simulink subsystem "Trajectory"  (R2021a)
settings: Solver=VariableStepAuto  StartTime=0.0  StopTime=10.0  RelTol=1e-3
undefined symbols (not defined in the file): DiscIntNeverNeededParam, MPC, mpc
libraries: robotlib x5, sharedtransform x2, robotcorelib x2, eeGeneralControl x1
settings Model: Creator=Lamarre  LastModifiedBy=lamarre
settings SolverCC: AlgebraicLoopSolver=TrustRegion
settings DebuggingCC: SFMachineParentedDataDiag=warning

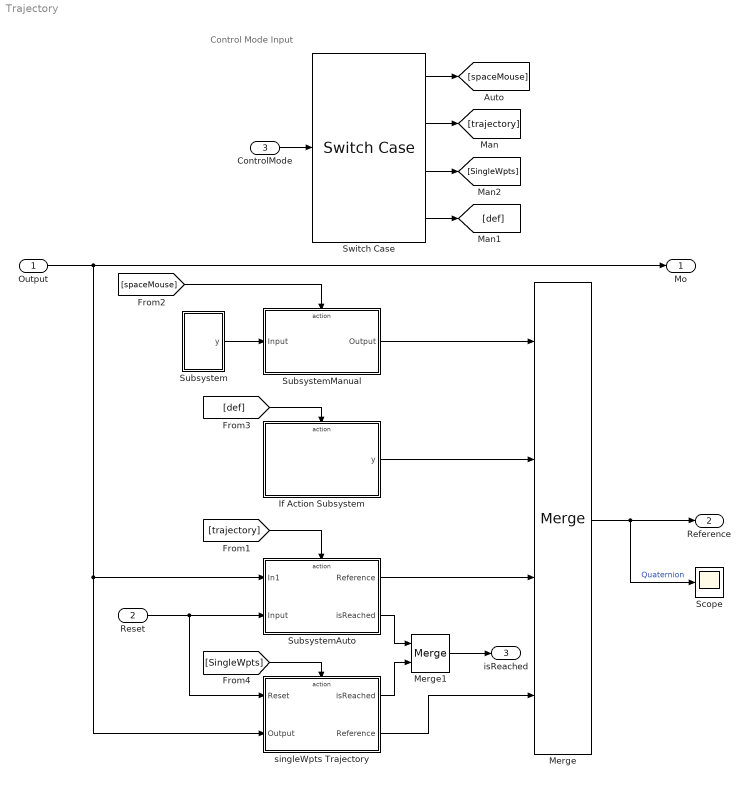
== system Trajectory ==
  note: Control Mode Input
  Output : Inport
  Reset : Inport  Port=2
  ControlMode : Inport  Port=3
  If Action Subsystem : Subsystem  TreatAsAtomicUnit=on
  Merge : Merge  Inputs=4
  Merge1 : Merge
  Scope : Scope
  Subsystem : Subsystem
  SubsystemAuto : Subsystem
  SubsystemManual : Subsystem
  Switch Case : SwitchCase  CaseConditions={mode.traj.SpaceMouseMode,mode.traj.trajMode, mode.traj.singleWpts,}
  singleWpts Trajectory : Subsystem
  Mo : Outport
  Reference : Outport  Port=2
  isReached : Outport  Port=3
  wires:
  Output/1 -> SubsystemAuto/1(In1), singleWpts Trajectory/2(Output), Mo/1
  Reset/1 -> SubsystemAuto/2(Input), singleWpts Trajectory/1(Reset)
  ControlMode/1 -> Switch Case/1
  [trajectory] -> SubsystemAuto/Action
  SubsystemManual/1(Output) -> Merge/1
  Subsystem/1(y) -> SubsystemManual/1(Input)
  [spaceMouse] -> SubsystemManual/Action
  Merge/1 -> Reference/1, Scope/1  "Quaternion"
  Switch Case/1 -> [spaceMouse]
  Switch Case/2 -> [trajectory]
  [def] -> If Action Subsystem/Action
  If Action Subsystem/1(y) -> Merge/2
  Switch Case/4 -> [def]
  Switch Case/3 -> [SingleWpts]
  [SingleWpts] -> singleWpts Trajectory/Action
  SubsystemAuto/2(isReached) -> Merge1/1
  Merge1/1 -> isReached/1
  singleWpts Trajectory/1("isReached ") -> Merge1/2
  singleWpts Trajectory/2("Reference ") -> Merge/4
  SubsystemAuto/1(Reference) -> Merge/3

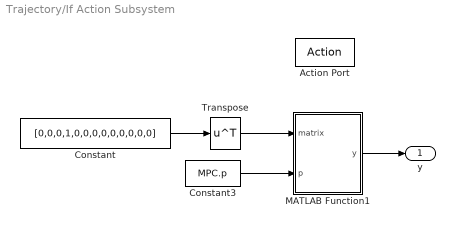
== system Trajectory/If Action Subsystem ==
  Action Port : ActionPort
  Constant : Constant  Value=[0,0,0,1,0,0,0,0,0,0,0,0,0]
  Constant3 : Constant  Value=MPC.p
  MATLAB Function1 : MATLAB Function  TreatAsAtomicUnit=on
  Transpose : Math  Operator=transpose  OutputSignalType=real  SaturateOnIntegerOverflow=on
  y : Outport
  wires:
  Constant/1 -> Transpose/1
  MATLAB Function1/1(y) -> y/1
  Constant3/1 -> MATLAB Function1/2(p)
  Transpose/1 -> MATLAB Function1/1(matrix)

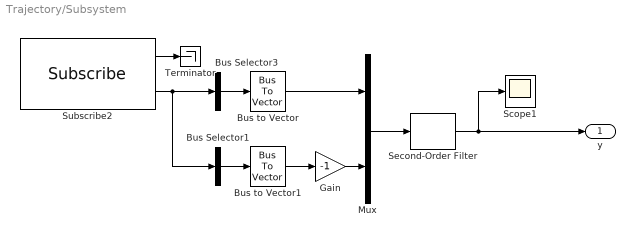
== system Trajectory/Subsystem ==
  Bus Selector1 : BusSelector  OutputSignals=Angular.X,Angular.Y,Angular.Z  OutputAsBus=on
  Bus Selector3 : BusSelector  OutputSignals=Linear.X,Linear.Y,Linear.Z  OutputAsBus=on
  Bus to Vector : BusToVector
  Bus to Vector1 : BusToVector
  Gain : Gain  Gain=-1
  Mux : Mux  Inputs=2
  Scope1 : Scope
  Second-Order Filter : eeGeneralControl/Second-Order Filter  FilterType=Low-pass  fn=wn_l  Zeta=zeta_l  Ts=1/25  A0=0  Ph0=0  f0=0  b0=0
      settings: SourceProductBaseCode=PS
  Subscribe2 : robotlib/Subscribe  topicSource=Specify your own  topic=/spacenav/twist  messageType=geometry_msgs/Twist  SampleTime=1/25  legacyBusStruct=off  messageQueueLength=2
  Terminator : Terminator
  y : Outport
  wires:
  Mux/1 -> Second-Order Filter/1
  Bus to Vector/1 -> Mux/1
  Gain/1 -> Mux/2
  Bus to Vector1/1 -> Gain/1
  Bus Selector1/1 -> Bus to Vector1/1
  Bus Selector3/1 -> Bus to Vector/1
  Subscribe2/1 -> Terminator/1
  Subscribe2/2 -> Bus Selector3/1, Bus Selector1/1
  Second-Order Filter/1 -> Scope1/1, y/1

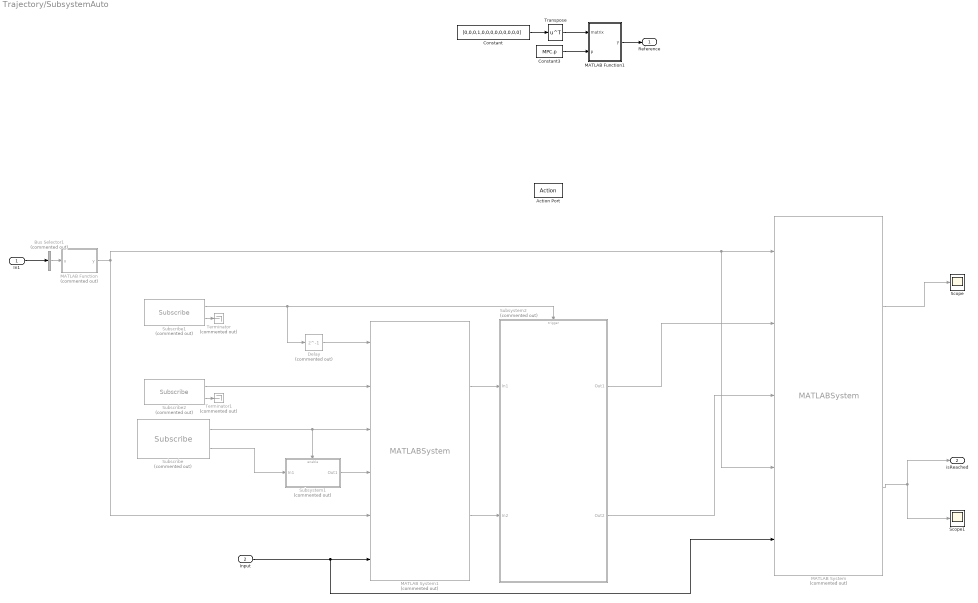
== system Trajectory/SubsystemAuto ==
  In1 : Inport
  Input : Inport  Port=2
  Action Port : ActionPort
  Bus Selector1 : BusSelector  Commented=on  OutputSignals=World Position,qS2W  OutputAsBus=on
  Constant : Constant  Value=[0,0,0,1,0,0,0,0,0,0,0,0,0]
  Constant3 : Constant  Value=MPC.p
  Delay : Delay  Commented=on  DelayLength=1
  MATLAB Function : MATLAB Function  Commented=on  TreatAsAtomicUnit=on
  MATLAB Function1 : MATLAB Function  TreatAsAtomicUnit=on
  MATLAB System : MATLABSystem  Commented=on  System=TrajectoryManager  SampleTime=mpc.Ts  OffsetTime=0  prediction=mpc.p  bufferSize=6001  linearConvergence=.2  quaternionConvergence=.1  TargetThreshold=3  SimulateUsing=Code generation
      mask Type: TrajectoryManager
      mask Display:
      | disp('TrajectoryManager');
      | port_label('input',1,'mesuredPose');
      | port_label('input',2,'poses');
      | port_label('input',3,'isNew');
      | port_label('input',4,'x0');
      | port_label('input',5,'reset');
      | port_label('output',1,'currentPose');
      | port_label('output',2,'isReached');
  MATLAB System1 : MATLABSystem  Commented=on  System=AddPose  buffSize=20  elementSize=8  SimulateUsing=Interpreted execution
      mask Type: AddPose
      mask Display:
      | disp('AddPose');
      | port_label('input',1,'compute');
      | port_label('input',2,'clearBuffer');
      | port_label('input',3,'isNew');
      | port_label('input',4,'waypoint');
      | port_label('input',5,'initCond');
      | port_label('input',6,'reset');
      | port_label('output',1,'waypoints');
      | port_label('output',2,'count');
  Scope : Scope
  Scope1 : Scope
  Subscribe : robotlib/Subscribe  Commented=on  topicSource=Specify your own  topic=proc_control/add_pose  messageType=sonia_common/AddPose  SampleTime=-1  legacyBusStruct=off  messageQueueLength=1
      link override SourceBlock: ROSTopic=/my_topic  ROSMessageType=geometry_msgs/Point  SLBusName=SL_Bus_Test_Traj_geometry_msgs_Point  ModelName=Test_Traj  BlockId=Sub_Test_Traj_124
  Subscribe1 : robotlib/Subscribe  Commented=on  topicSource=Specify your own  topic=/proc_control/compute_trajectory  messageType=std_msgs/Bool  SampleTime=-1  legacyBusStruct=off  messageQueueLength=1
  Subscribe2 : robotlib/Subscribe  Commented=on  topicSource=Specify your own  topic=/proc_control/clear_waypoints  messageType=std_msgs/Bool  SampleTime=-1  legacyBusStruct=off  messageQueueLength=1
  Subsystem1 : Subsystem  Commented=on
  Subsystem2 : Subsystem  Commented=on
  Terminator : Terminator  Commented=on
  Terminator1 : Terminator  Commented=on
  Transpose : Math  Operator=transpose  OutputSignalType=real  SaturateOnIntegerOverflow=on
  Reference : Outport
  isReached : Outport  Port=2
  wires:
  Constant/1 -> Transpose/1
  Constant3/1 -> MATLAB Function1/2(p)
  Transpose/1 -> MATLAB Function1/1(matrix)
  MATLAB Function1/1(y) -> Reference/1
  Subscribe2/2 -> Terminator1/1
  Subscribe1/2 -> Terminator/1
  Input/1 -> MATLAB System1/6, MATLAB System/5
  Subscribe2/1 -> MATLAB System1/2
  MATLAB Function/1(y) -> MATLAB System1/5, MATLAB System/1, MATLAB System/4
  Subscribe/1 -> MATLAB System1/3, Subsystem1/Enable
  MATLAB System/1 -> Scope/1
  Subsystem2/1(Out1) -> MATLAB System/2
  Subsystem2/2(Out2) -> MATLAB System/3
  Subscribe/2 -> Subsystem1/1(In1)
  Subsystem1/1(Out1) -> MATLAB System1/4
  In1/1 -> Bus Selector1/1
  MATLAB System/2 -> Scope1/1, isReached/1
  MATLAB System1/2 -> Subsystem2/2(In2)
  Subscribe1/1 -> Delay/1, Subsystem2/Trigger
  Bus Selector1/1 -> MATLAB Function/1(u)
  MATLAB System1/1 -> Subsystem2/1(In1)
  Delay/1 -> MATLAB System1/1

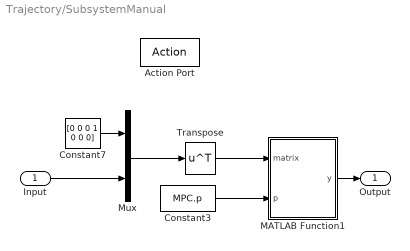
== system Trajectory/SubsystemManual ==
  Input : Inport
  Action Port : ActionPort
  Constant3 : Constant  Value=MPC.p
  Constant7 : Constant  Value=[0 0 0 1 0 0 0]
  MATLAB Function1 : MATLAB Function  TreatAsAtomicUnit=on
  Mux : Mux  Inputs=2
  Transpose : Math  Operator=transpose  OutputSignalType=real  SaturateOnIntegerOverflow=on
  Output : Outport
  wires:
  MATLAB Function1/1(y) -> Output/1
  Mux/1 -> Transpose/1
  Constant3/1 -> MATLAB Function1/2(p)
  Transpose/1 -> MATLAB Function1/1(matrix)
  Input/1 -> Mux/2
  Constant7/1 -> Mux/1

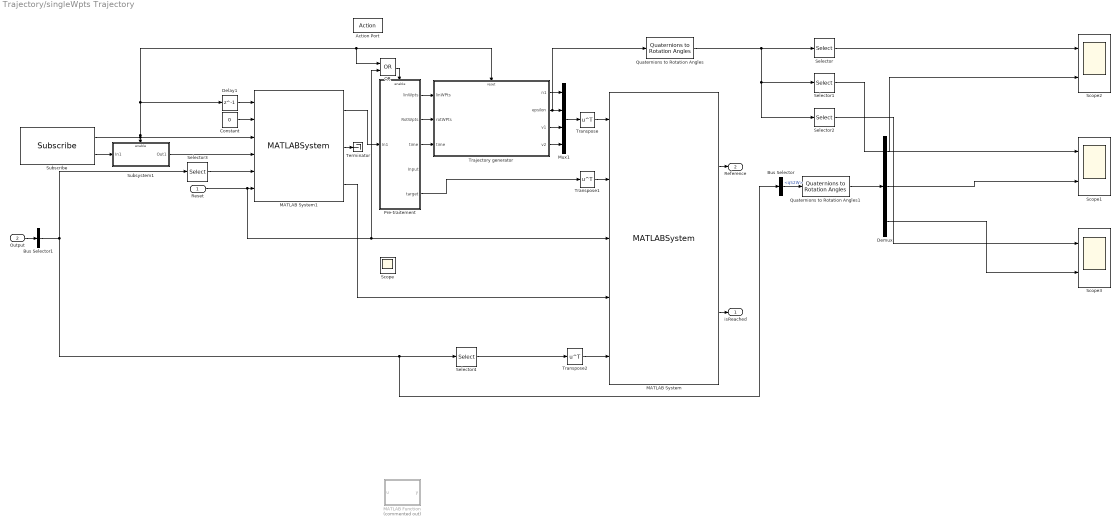
== system Trajectory/singleWpts Trajectory ==
  Reset : Inport
  Output : Inport  Port=2
  Action Port : ActionPort  InitializeStates=reset
  Bus Selector : BusSelector  OutputSignals=qS2W
  Bus Selector1 : BusSelector  OutputSignals=World Position,qS2W,Body Velocity,Angular Rate  OutputAsBus=on
  Constant : Constant  Value=0
  Delay1 : Delay  DelayLength=1
  Demux : Demux  Outputs=3
  MATLAB Function : MATLAB Function  Commented=on  TreatAsAtomicUnit=on
  MATLAB System : MATLABSystem  System=TrajectoryManager  SampleTime=MPC.Ts  OffsetTime=0  prediction=MPC.p  bufferSize=6001  linearConvergence=.25  quaternionConvergence=.22  TargetThreshold=2  SimulateUsing=Code generation
      mask Type: TrajectoryManager
      mask Display:
      | disp('TrajectoryManager');
      | port_label('input',1,'poses');
      | port_label('input',2,'target');
      | port_label('input',3,'reset');
      | port_label('input',4,'x0');
      | port_label('input',5,'mesuredPose');
      | port_label('output',1,'currentPose');
      | port_label('output',2,'isReached');
  MATLAB System1 : MATLABSystem  System=AddPose  buffSize=2  elementSize=9  SimulateUsing=Code generation
      mask Type: AddPose
      mask Display:
      | disp('AddPose');
      | port_label('input',1,'compute');
      | port_label('input',2,'clearBuffer');
      | port_label('input',3,'isNew');
      | port_label('input',4,'waypoint');
      | port_label('input',5,'xk');
      | port_label('input',6,'reset');
      | port_label('output',1,'waypoints');
      | port_label('output',2,'count');
      | port_label('output',3,'initCond');
  Mux1 : Mux
  OR : Logic  Operator=OR  AllPortsSameDT=off  OutDataTypeStr=boolean
  Pre-traitement : Subsystem
  Quaternions to Rotation Angles : sharedtransform/Quaternions to Rotation Angles  rotationOrder=ZYX  aMode=aMode
      settings: SourceProductBaseCode=AE,PW,DR,MT,UV,VE
  Quaternions to Rotation Angles1 : sharedtransform/Quaternions to Rotation Angles  rotationOrder=ZYX  aMode=aMode
      settings: SourceProductBaseCode=AE,PW,DR,MT,UV,VE
  Scope : Scope
  Scope1 : Scope  NumInputPorts=2
  Scope2 : Scope  NumInputPorts=2
  Scope3 : Scope  NumInputPorts=2
  Selector : Selector  InputPortWidth=3  IndexOptions=Index vector (dialog)  Indices=[1]  OutputSizes=1
  Selector1 : Selector  InputPortWidth=3  IndexOptions=Index vector (dialog)  Indices=[2]  OutputSizes=1
  Selector2 : Selector  InputPortWidth=3  IndexOptions=Index vector (dialog)  Indices=[3]  OutputSizes=1
  Selector3 : Selector  InputPortWidth=13  IndexOptions=Index vector (dialog)  Indices=[1:7]  OutputSizes=1
  Selector4 : Selector  InputPortWidth=13  IndexOptions=Index vector (dialog)  Indices=[1:13]  OutputSizes=1
  Subscribe : robotlib/Subscribe  topicSource=Specify your own  topic=proc_control/add_pose  messageType=sonia_common/AddPose  SampleTime=-1  legacyBusStruct=off  messageQueueLength=1
      link override SourceBlock: ROSTopic=/my_topic  ROSMessageType=geometry_msgs/Point  SLBusName=SL_Bus_Test_Traj_geometry_msgs_Point  ModelName=Test_Traj  BlockId=Sub_Test_Traj_124
  Subsystem1 : Subsystem
  Terminator : Terminator
  Trajectory generator : Subsystem
  Transpose : Math  Operator=transpose  SaturateOnIntegerOverflow=on
  Transpose1 : Math  Operator=transpose  SaturateOnIntegerOverflow=on
  Transpose2 : Math  Operator=transpose  SaturateOnIntegerOverflow=on
  "isReached " : Outport
  "Reference " : Outport  Port=2
  wires:
  Bus Selector/1 -> Quaternions to Rotation Angles1/1  "<qS2W>"
  Quaternions to Rotation Angles1/1 -> Demux/1
  Quaternions to Rotation Angles/1 -> Selector/1, Selector1/1, Selector2/1
  Trajectory generator/2(epsilon) -> Mux1/2, Quaternions to Rotation Angles/1
  Transpose2/1 -> MATLAB System/5
  MATLAB System1/3 -> MATLAB System/4
  Transpose1/1 -> MATLAB System/2
  Pre-traitement/5(target) -> Transpose1/1
  Demux/3 -> Scope3/2
  Demux/2 -> Scope1/2
  Demux/1 -> Scope2/2
  Selector2/1 -> Scope3/1
  Selector1/1 -> Scope1/1
  Selector/1 -> Scope2/1
  Selector3/1 -> MATLAB System1/5
  Transpose/1 -> MATLAB System/1
  Trajectory generator/1(n1) -> Mux1/1
  Trajectory generator/4(v2) -> Mux1/4
  Trajectory generator/3(v1) -> Mux1/3
  Selector4/1 -> Transpose2/1
  Mux1/1 -> Transpose/1
  Bus Selector1/1 -> Selector3/1, Bus Selector/1, Selector4/1
  MATLAB System/2 -> "isReached "/1
  MATLAB System1/1 -> Pre-traitement/1(In1)
  Reset/1 -> MATLAB System1/6, MATLAB System/3, OR/2
  Output/1 -> Bus Selector1/1
  OR/1 -> Pre-traitement/Enable
  Delay1/1 -> MATLAB System1/1
  MATLAB System/1 -> "Reference "/1
  Pre-traitement/3(time) -> Trajectory generator/3(time)
  Pre-traitement/2(RotWpts) -> Trajectory generator/2(rotWPts)
  Pre-traitement/1(linWpts) -> Trajectory generator/1(linWPts)
  MATLAB System1/2 -> Terminator/1
  Constant/1 -> MATLAB System1/2
  Subsystem1/1(Out1) -> MATLAB System1/4
  Subscribe/1 -> MATLAB System1/3, Subsystem1/Enable, Delay1/1, OR/1, Trajectory generator/Reset
  Subscribe/2 -> Subsystem1/1(In1)

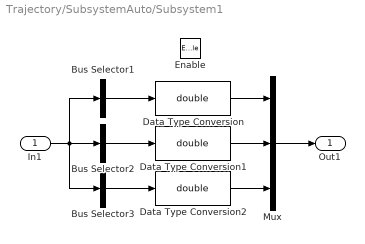
== system Trajectory/SubsystemAuto/Subsystem1 ==
  In1 : Inport
  Enable : EnablePort
  Bus Selector1 : BusSelector  OutputSignals=Position.X,Position.Y,Position.Z,Orientation.Z,Orientation.Y,Orientation.X  OutputAsBus=on
  Bus Selector2 : BusSelector  OutputSignals=Frame,Speed  OutputAsBus=on
  Bus Selector3 : BusSelector  OutputSignals=Fine  OutputAsBus=on
  Data Type Conversion : DataTypeConversion  OutDataTypeStr=double  LockScale=on
  Data Type Conversion1 : DataTypeConversion  OutDataTypeStr=double  LockScale=on
  Data Type Conversion2 : DataTypeConversion  OutDataTypeStr=double  LockScale=on
  Mux : Mux  Inputs=3
  Out1 : Outport
  wires:
  Mux/1 -> Out1/1
  Data Type Conversion2/1 -> Mux/3
  Data Type Conversion1/1 -> Mux/2
  Data Type Conversion/1 -> Mux/1
  Bus Selector3/1 -> Data Type Conversion2/1
  Bus Selector2/1 -> Data Type Conversion1/1
  In1/1 -> Bus Selector2/1, Bus Selector3/1, Bus Selector1/1
  Bus Selector1/1 -> Data Type Conversion/1

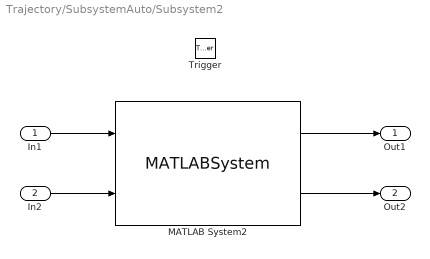
== system Trajectory/SubsystemAuto/Subsystem2 ==
  In1 : Inport
  In2 : Inport  Port=2
  Trigger : TriggerPort  VariantControl=Variant  PortDimensions=1
  MATLAB System2 : MATLABSystem  System=TrajectoryGenerator  avanceRapide=[1 1 .3 .1 .1 .1 .1]  avancePrecision=[.3 .3 .1 .05 .05 .05 .05]  accRapide=[0.2 0.2 0.1 .02 .02 .02 .02];  accPrecision=0.1  Ts=0.25  bufferSize=1000  SimulateUsing=Interpreted execution
      mask Type: TrajectoryGenerator
      mask Display:
      | disp('TrajectoryGenerator');
      | port_label('input',1,'wpts');
      | port_label('input',2,'wpt_count');
      | port_label('output',1,'pose');
      | port_label('output',2,'new');
  Out1 : Outport
  Out2 : Outport  Port=2
  wires:
  MATLAB System2/2 -> Out2/1
  MATLAB System2/1 -> Out1/1
  In2/1 -> MATLAB System2/2
  In1/1 -> MATLAB System2/1

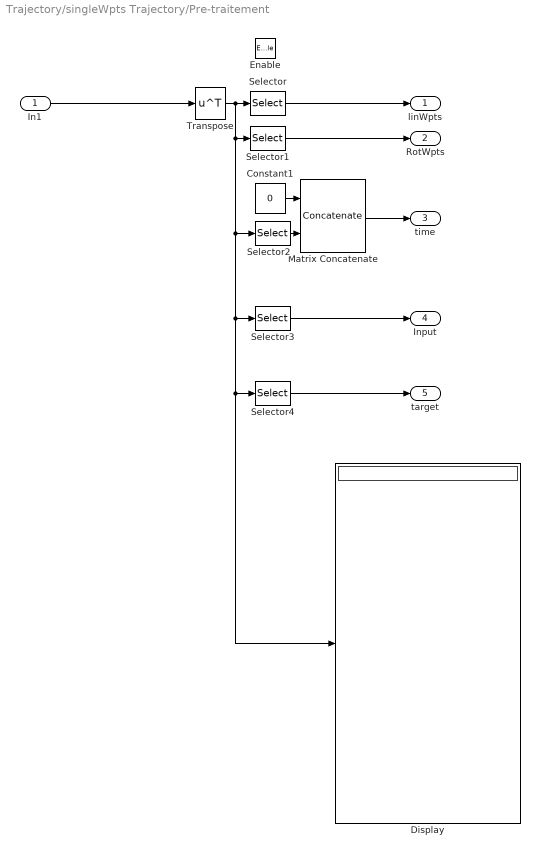
== system Trajectory/singleWpts Trajectory/Pre-traitement ==
  In1 : Inport
  Enable : EnablePort
  Constant1 : Constant  Value=0
  Display : Display
  Matrix Concatenate : Concatenate  Mode=Multidimensional array
  Selector : Selector  NumberOfDimensions=2  InputPortWidth=3  IndexOptions=Index vector (dialog),Index vector (dialog)  Indices=[1:3],[1:2]  OutputSizes=1,1
  Selector1 : Selector  NumberOfDimensions=2  InputPortWidth=3  IndexOptions=Index vector (dialog),Index vector (dialog)  Indices=[4:7],[1:2]  OutputSizes=1,1
  Selector2 : Selector  NumberOfDimensions=2  InputPortWidth=3  IndexOptions=Index vector (dialog),Index vector (dialog)  Indices=[8],[2]  OutputSizes=1,1
  Selector3 : Selector  NumberOfDimensions=2  InputPortWidth=3  IndexOptions=Index vector (dialog),Index vector (dialog)  Indices=[9],[2]  OutputSizes=1,1
  Selector4 : Selector  NumberOfDimensions=2  InputPortWidth=3  IndexOptions=Index vector (dialog),Index vector (dialog)  Indices=[1:7],[2]  OutputSizes=1,1
  Transpose : Math  Operator=transpose  SaturateOnIntegerOverflow=on
  linWpts : Outport
  RotWpts : Outport  Port=2
  time : Outport  Port=3
  Input : Outport  Port=4
  target : Outport  Port=5
  wires:
  Selector4/1 -> target/1
  Selector3/1 -> Input/1
  Selector1/1 -> RotWpts/1
  Matrix Concatenate/1 -> time/1
  Constant1/1 -> Matrix Concatenate/1
  Selector2/1 -> Matrix Concatenate/2
  In1/1 -> Transpose/1
  Transpose/1 -> Selector/1, Selector1/1, Display/1, Selector4/1, Selector3/1, Selector2/1
  Selector/1 -> linWpts/1

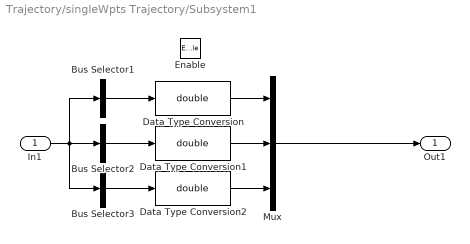
== system Trajectory/singleWpts Trajectory/Subsystem1 ==
  In1 : Inport
  Enable : EnablePort
  Bus Selector1 : BusSelector  OutputSignals=Position.X,Position.Y,Position.Z,Orientation.Z,Orientation.Y,Orientation.X  OutputAsBus=on
  Bus Selector2 : BusSelector  OutputSignals=Frame,Speed  OutputAsBus=on
  Bus Selector3 : BusSelector  OutputSignals=Fine  OutputAsBus=on
  Data Type Conversion : DataTypeConversion  OutDataTypeStr=double  LockScale=on
  Data Type Conversion1 : DataTypeConversion  OutDataTypeStr=double  LockScale=on
  Data Type Conversion2 : DataTypeConversion  OutDataTypeStr=double  LockScale=on
  Mux : Mux  Inputs=3
  Out1 : Outport
  wires:
  Mux/1 -> Out1/1
  Data Type Conversion2/1 -> Mux/3
  Data Type Conversion1/1 -> Mux/2
  Data Type Conversion/1 -> Mux/1
  Bus Selector3/1 -> Data Type Conversion2/1
  Bus Selector2/1 -> Data Type Conversion1/1
  In1/1 -> Bus Selector2/1, Bus Selector3/1, Bus Selector1/1
  Bus Selector1/1 -> Data Type Conversion/1

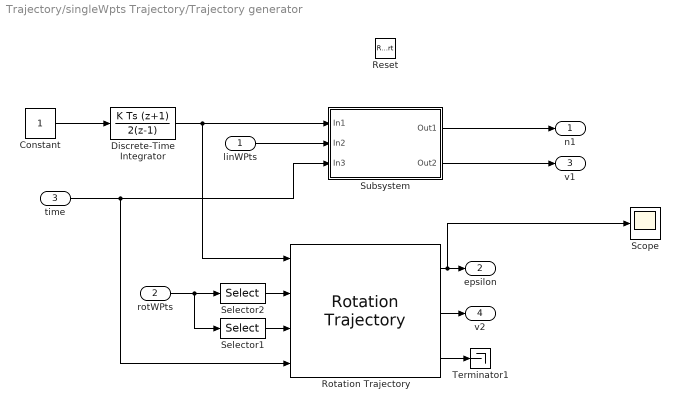
== system Trajectory/singleWpts Trajectory/Trajectory generator ==
  linWPts : Inport
  rotWPts : Inport  Port=2
  time : Inport  Port=3
  Reset : ResetPort  DisableCoverage=on
  Constant : Constant
  Discrete-Time Integrator : DiscreteIntegrator  IntegratorMethod=Integration: Trapezoidal  SampleTime=-1  ICPrevOutput=DiscIntNeverNeededParam  ICPrevScaledInput=DiscIntNeverNeededParam
  Rotation Trajectory : robotcorelib/Rotation Trajectory  WaypointFormat=Quaternion  WaypointSource=External  R0=[ 1, 0, 0, 0 ]'  RF=[ 0, 0, 1, 0 ]'  TimeInterval=[ 0, 1 ]  CustomTimeScaling=off  ParameterSource=Internal  TSTime=0:0.1:1  TimeScaling=[ 0:0.1:1; ones( 1, 11 ); zeros( 1, 11 ) ]  SimulateUsing=Code generation
      settings: SourceProductBaseCode=NV,RO,RR,UV
  Scope : Scope
  Selector1 : Selector  NumberOfDimensions=2  InputPortWidth=3  IndexOptions=Index vector (dialog),Index vector (dialog)  Indices=[1:4],2  OutputSizes=1,1
  Selector2 : Selector  NumberOfDimensions=2  InputPortWidth=3  IndexOptions=Index vector (dialog),Index vector (dialog)  Indices=[1:4],1  OutputSizes=1,1
  Subsystem : Subsystem
  Terminator1 : Terminator
  n1 : Outport
  epsilon : Outport  Port=2
  v1 : Outport  Port=3
  v2 : Outport  Port=4
  wires:
  Rotation Trajectory/2 -> v2/1
  Subsystem/2(Out2) -> v1/1
  Subsystem/1(Out1) -> n1/1
  Rotation Trajectory/1 -> epsilon/1, Scope/1
  Selector1/1 -> Rotation Trajectory/3
  Selector2/1 -> Rotation Trajectory/2
  rotWPts/1 -> Selector2/1, Selector1/1
  Rotation Trajectory/3 -> Terminator1/1
  time/1 -> Subsystem/3(In3), Rotation Trajectory/4
  linWPts/1 -> Subsystem/2(In2)
  Discrete-Time Integrator/1 -> Subsystem/1(In1), Rotation Trajectory/1
  Constant/1 -> Discrete-Time Integrator/1

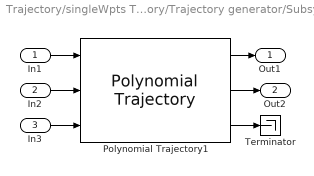
== system Trajectory/singleWpts Trajectory/Trajectory generator/Subsystem ==
  In1 : Inport
  In2 : Inport  Port=2
  In3 : Inport  Port=3
  Polynomial Trajectory1 : robotcorelib/Polynomial Trajectory  WaypointSource=External  Waypoints=wayPoints  TimePoints=[ 0, 1, 2, 3, 4 ]  TimeInterval=[0,5]  Method=Cubic Polynomial  ParameterSource=Internal  VelocityBoundaryCondition=zeros( 3, 2 )  AccelerationBoundaryCondition=zeros( 2, 5 )  SimulateUsing=Code generation
  Terminator : Terminator
  Out1 : Outport
  Out2 : Outport  Port=2
  wires:
  Polynomial Trajectory1/2 -> Out2/1
  In3/1 -> Polynomial Trajectory1/3
  Polynomial Trajectory1/1 -> Out1/1
  Polynomial Trajectory1/3 -> Terminator/1
  In1/1 -> Polynomial Trajectory1/1
  In2/1 -> Polynomial Trajectory1/2

== matlab function Trajectory/If Action Subsystem/MATLAB Function1 ==
  data: matrix input; y output size=[10 13]; p input
function y = fcn(matrix,p)
matrix(10)=-matrix(10);
y = repmat(matrix,10,1);

== matlab function Trajectory/SubsystemManual/MATLAB Function1 ==
  data: matrix input; y output size=[10 13]; p input
function y = fcn(matrix,p)
%matrix(10)=-matrix(10);
y = repmat(matrix,10,1);

== matlab function Trajectory/singleWpts Trajectory/MATLAB Function ==
  data: y output size=[1,13]; u input size=[1,13]
function y = fcn(u)

y = u;

== matlab function Trajectory/SubsystemAuto/MATLAB Function1 ==
  data: matrix input; y output size=[10 13]; p input
function y = fcn(matrix,p)
matrix(10)=-matrix(10);
y = repmat(matrix,10,1);

== matlab function Trajectory/SubsystemAuto/MATLAB Function ==
  data: u input size=[1,7]; y output size=[1,7]
function y = fcn(u)

y = u;
